simulink model "Nivel_tanque_corregido"  (R2024a)
settings: Solver=FixedStepAuto  StartTime=0.0  StopTime=inf  RelTol=1e-3
undefined symbols (not defined in the file): daq
libraries: daqlib x6, fuzblock x1
settings Model: Creator=nuevo  LastModifiedBy=USER
settings SolverCC: AlgebraicLoopSolver=TrustRegion
settings DataIOCC: LimitDataPoints=on  SaveFormat=Array  SignalLoggingSaveFormat=ModelDataLogs  ReturnWorkspaceOutputs=off
settings OptimizationCC: ExpressionDepthLimit=2147483647  LifeSpan=inf
settings DebuggingCC: UnderspecifiedInitializationDetection=Classic  MergeDetectMultiDrivingBlocksExec=none  SolverPrmCheckMsg=warning  FcnCallInpInsideContextMsg=warning  UnconnectedInputMsg=warning  UnconnectedOutputMsg=warning  UnconnectedLineMsg=warning  StateNameClashWarn=warning  SFUnexpectedBacktrackingDiag=warning  SFNoUnconditionalDefaultTransitionDiag=warning  SFExecutionAtInitializationDiag=none  ArithmeticOperatorsInVariantConditions=warning
settings HardwareCC: ProdBitPerPointer=32  ProdBitPerSizeT=32  ProdBitPerPtrDiffT=32  ProdLargestAtomicFloat=None  ProdIntDivRoundTo=Undefined  ProdEndianess=Unspecified  ProdWordSize=32  ProdHWDeviceType=32-bit Generic
settings ModelReferenceCC: EnableRefExpFcnMdlSchedulingChecks=on  PropagateSignalLabelsOutOfModel=off
settings SFSimCC: SimUseLocalCustomCode=off  CustomCodeUndefinedFunction=UseInterfaceOnly
settings RTWCC: RTWUseLocalCustomCode=off  GPUComputeCapability=3.5  DLArmComputeVersion=19.05
settings CodeAppCC: StateflowObjectComments=on
settings GRTTargetCC: TargetLangStandard=C89/C90 (ANSI)  CombineOutputUpdateFcns=off  GRTInterface=on
settings ConfigComp: CovMetricSettings=dw  CovSaveCumulativeToWorkspaceVar=on  CovSaveSingleToWorkspaceVar=on  CovExternalEMLEnable=off

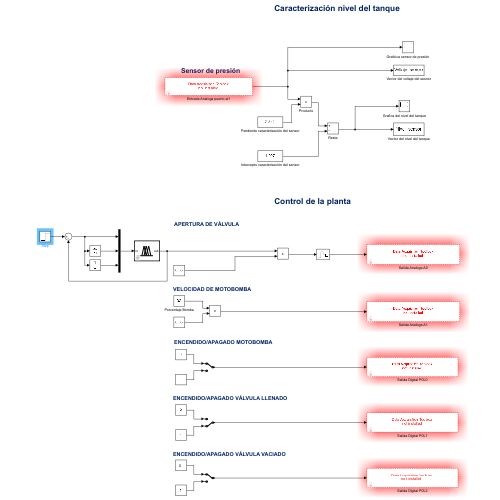
[thumbnail: Simulink's stored preview of the top-level diagram]
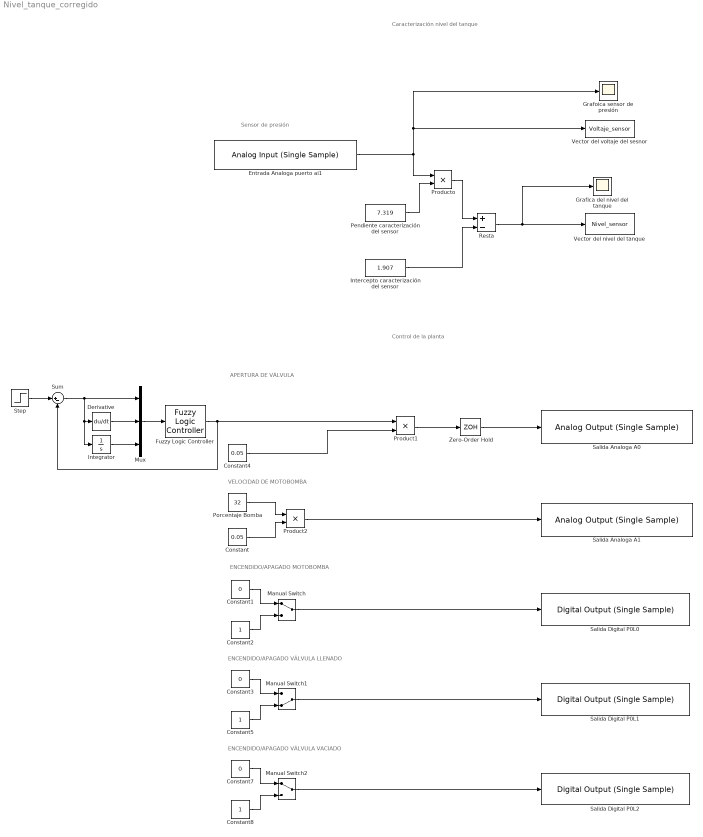
== system Nivel_tanque_corregido ==
  note: Caracterización nivel del tanque
  note: Sensor de presión
  note: Control de la planta
  note: APERTURA DE VÁLVULA
  note: ENCENDIDO/APAGADO MOTOBOMBA
  note: VELOCIDAD DE MOTOBOMBA
  note: ENCENDIDO/APAGADO VÁLVULA LLENADO
  note: ENCENDIDO/APAGADO VÁLVULA VACIADO
  Constant : Constant  Value=0.05
  Constant1 : Constant  Value=0  OutDataTypeStr=boolean
  Constant2 : Constant  OutDataTypeStr=boolean
  Constant3 : Constant  Value=0  OutDataTypeStr=boolean
  Constant4 : Constant  Value=0.05
  Constant5 : Constant  OutDataTypeStr=boolean
  Constant7 : Constant  Value=0  OutDataTypeStr=boolean
  Constant8 : Constant  OutDataTypeStr=boolean
  Derivative : Derivative
  Entrada Analoga puerto ai1 : daqlib/Analog Input (Single Sample)  DeviceMenu=ni Dev1 (USB-6009)  Device=ni Dev1 (USB-6009)  ObjConstructor=daq.createSession('ni')  BlockSampleTime=0.04  NChannelsSelected=1  Channels=0$ai0$$Dev1$1$8$2$1$#1$ai1$$Dev1$1$8$2$1$#0$ai2$$Dev1$1$8$2$1$#0$ai3$$Dev1$1$8$2$1$#0$ai4$$Dev1$1$7$1$1$#0$ai5$$Dev1$1$7$1$1$#0$ai6$$Dev1$1$7$1$1$#0$ai7$$Dev1$1$7$1$1$#  NPorts=1 for all channels  OutputTimestamp=off
  Fuzzy Logic Controller : fuzblock/Fuzzy Logic  Controller  FIS='planta_fuzzy.fis'  OutputSampleNumber=101  DataType=double  FuzzifiedInputs=off  RuleFiringStrengths=off  RuleOutputs=off  AggregatedOutputs=off  SimulateUsing=Interpreted execution  OutOfRangeInputValueMessage=warning  NoRuleFiredMessage=warning  EmptyOutputFuzzySetMessage=warning
  Grafica del nivel del tanque : Scope
  Grafoica sensor de presión : Scope
  Integrator : Integrator
  Intercepto caracterización del sensor : Constant  Value=1.907
  Manual Switch : ManualSwitch
  Manual Switch1 : ManualSwitch  CurrentSetting=0
  Manual Switch2 : ManualSwitch
  Mux : Mux  Inputs=3
  Pendiente caracterización del sensor : Constant  Value=7.319
  Porcentaje Bomba : Constant  Value=32
  Product1 : Product  RndMeth=Zero
  Product2 : Product  RndMeth=Zero
  Producto : Product  RndMeth=Zero
  Resta : Sum  Inputs=+-
  Salida Analoga A0 : daqlib/Analog Output (Single Sample)  DeviceMenu=ni Dev1 (USB-6009)  Device=ni Dev1 (USB-6009)  ObjConstructor=daq.createSession('ni')  NChannelsSelected=1  Channels=1$ao0$$Dev1$1$1$N/A$#0$ao1$$Dev1$1$1$N/A$#  NPorts=1 for all channels  BlockSampleTime=1
  Salida Analoga A1 : daqlib/Analog Output (Single Sample)  DeviceMenu=ni Dev1 (USB-6009)  Device=ni Dev1 (USB-6009)  ObjConstructor=daq.createSession('ni')  NChannelsSelected=1  Channels=0$ao0$$Dev1$1$1$N/A$#1$ao1$$Dev1$1$1$N/A$#  NPorts=1 for all channels  BlockSampleTime=1
  Salida Digital P0L0 : daqlib/Digital Output (Single Sample)  DeviceMenu=ni Dev1 (USB-6009)  Device=ni Dev1 (USB-6009)  ObjConstructor=daq.createSession('ni')  BlockSampleTime=1  IsDigitalInput=off  NLinesSelected=1  Lines=1$port0/line0$$Dev1$#0$port0/line1$$Dev1$#0$port0/line2$$Dev1$#0$port0/line3$$Dev1$#0$port0/line4$$Dev1$#0$port0/line5$$Dev1$#0$port0/line6$$Dev1$#0$port0/line7$$Dev1$#0$port1/line0$$Dev1$#0$port1/line1$$Dev1$#0$port1/line2$$Dev1$#0$port1/line3$$Dev1$#  NPorts=1 for all lines
  Salida Digital P0L1 : daqlib/Digital Output (Single Sample)  DeviceMenu=ni Dev1 (USB-6009)  Device=ni Dev1 (USB-6009)  ObjConstructor=daq.createSession('ni')  BlockSampleTime=1  IsDigitalInput=off  NLinesSelected=1  Lines=0$port0/line0$$Dev1$#1$port0/line1$$Dev1$#0$port0/line2$$Dev1$#0$port0/line3$$Dev1$#0$port0/line4$$Dev1$#0$port0/line5$$Dev1$#0$port0/line6$$Dev1$#0$port0/line7$$Dev1$#0$port1/line0$$Dev1$#0$port1/line1$$Dev1$#0$port1/line2$$Dev1$#0$port1/line3$$Dev1$#  NPorts=1 for all lines
  Salida Digital P0L2 : daqlib/Digital Output (Single Sample)  DeviceMenu=ni Dev1 (USB-6009)  Device=ni Dev1 (USB-6009)  ObjConstructor=daq.createSession('ni')  BlockSampleTime=1  IsDigitalInput=off  NLinesSelected=1  Lines=0$port0/line0$$Dev1$#0$port0/line1$$Dev1$#1$port0/line2$$Dev1$#0$port0/line3$$Dev1$#0$port0/line4$$Dev1$#0$port0/line5$$Dev1$#0$port0/line6$$Dev1$#0$port0/line7$$Dev1$#0$port1/line0$$Dev1$#0$port1/line1$$Dev1$#0$port1/line2$$Dev1$#0$port1/line3$$Dev1$#  NPorts=1 for all lines
  Step : Step  After=30  SampleTime=0
  Sum : Sum  Inputs=|+-
  Vector del nivel del tanque : ToWorkspace  VariableName=Nivel_sensor  SampleTime=0.04
      settings: Save2DSignal=2-D array (concatenate along first dimension)
  Vector del voltaje del sesnor : ToWorkspace  VariableName=Voltaje_sensor  SampleTime=0.04
      settings: Save2DSignal=2-D array (concatenate along first dimension)
  Zero-Order Hold : ZeroOrderHold
  wires:
  Pendiente caracterización del sensor/1 -> Producto/2
  Producto/1 -> Resta/1
  Intercepto caracterización del sensor/1 -> Resta/2
  Resta/1 -> Grafica del nivel del tanque/1, Vector del nivel del tanque/1
  Entrada Analoga puerto ai1/1 -> Vector del voltaje del sesnor/1, Grafoica sensor de presión/1, Producto/1
  Manual Switch2/1 -> Salida Digital P0L2/1
  Constant4/1 -> Product1/2
  Porcentaje Bomba/1 -> Product2/1
  Constant/1 -> Product2/2
  Constant2/1 -> Manual Switch/2
  Constant3/1 -> Manual Switch1/1
  Manual Switch1/1 -> Salida Digital P0L1/1
  Constant7/1 -> Manual Switch2/1
  Manual Switch/1 -> Salida Digital P0L0/1
  Constant8/1 -> Manual Switch2/2
  Constant5/1 -> Manual Switch1/2
  Constant1/1 -> Manual Switch/1
  Product2/1 -> Salida Analoga A1/1
  Product1/1 -> Zero-Order Hold/1
  Zero-Order Hold/1 -> Salida Analoga A0/1
  Mux/1 -> Fuzzy Logic Controller/1
  Sum/1 -> Integrator/1, Derivative/1, Mux/1
  Step/1 -> Sum/1
  Integrator/1 -> Mux/3
  Derivative/1 -> Mux/2
  Fuzzy Logic Controller/1 -> Sum/2, Product1/1
